simulink model "IL86_NEW_17a"  (R2021b)
settings: Solver=ode1  StartTime=0.0  StopTime=100  FixedStep=0.001  RelTol=1e-3  EnableMultiTasking=on
InitFcn:
  | INIT
values from neighbouring files (symbols this model uses):
  CBN0 = [XB0(1) XB0(2) XB0(3); XB0(4) XB0(5) XB0(6); XB0(7) XB0(8) XB0(9)]    [INIT.m]
  HTR = 500.0    (= 500)    [INIT.m]
  PAR = [1.700E05    5            8.400E06     3.000E07     2.300E07       -0.700E06    0.00E00      0.093E00     0.006E00     0.145E-01       0.586E-01  -0.518E-01    0.876E-01   -1.920E-04    8.110E-05       0.000E00   -2.330E-03    5.020E-04   -1.340E-05    0.515E-01      -3.215E-02   5.300E-04   -0.185E-01   -0.465E-01   -1.290E01       -5.000E00   -0.152E-01   -0.344E-02   -0.064E-02    5.200E-05     ...(+300 chars)    [INITLA.m]
  T_AIL = 1.0/20.2    (= 0.049504950495)    [INITLA.m]
  T_ELEV = 0.1    [INITLA.m]
  T_RUD = 1.0/20.2    (= 0.049504950495)    [INITLA.m]
  T_THROTTLE = 5.0    (= 5)    [INITLA.m]
  TGLIDE = 100.0    (= 100)    [INIT.m]
  THETATR = 0.0    (= 0)    [INIT.m]
  U0_GLIDE = [BAL(1);BAL(3);BAL(4);BAL(5)]    [INIT.m]
  U0_HORIZ = [BAL(1);BAL(3);BAL(4);BAL(5)]    [INIT.m]
  VTR = 80.0    (= 80)    [INIT.m]
  X0 = [Vx1,Vy1,Vz1,Wx1,Wy1,Wz1,GAM,PSI,TET,L,H,Z,FI,LAMD,d,deltaT,deltaV,deltaN,deltaE,Vwx1,Vwy1,Vwz1,HFL,EPS,X1]    [INTSTATE.m]
undefined symbols (not defined in the file or in its folder): BAL
settings Model: Creator=XINGAU  LastModifiedBy=peter
settings SolverCC: AlgebraicLoopSolver=TrustRegion
settings DataIOCC: LimitDataPoints=on  SaveFormat=Array  ReturnWorkspaceOutputs=off
settings OptimizationCC: ExpressionDepthLimit=2147483647  LifeSpan=inf
settings DebuggingCC: UnderspecifiedInitializationDetection=Classic  MergeDetectMultiDrivingBlocksExec=none  SolverPrmCheckMsg=warning  MultiTaskRateTransMsg=warning  StateNameClashWarn=warning  SFUnexpectedBacktrackingDiag=warning  SFNoUnconditionalDefaultTransitionDiag=warning  SFExecutionAtInitializationDiag=none  SFMachineParentedDataDiag=warning  ArithmeticOperatorsInVariantConditions=warning
settings HardwareCC: ProdBitPerPointer=32  ProdBitPerSizeT=32  ProdBitPerPtrDiffT=32  ProdLargestAtomicFloat=None  ProdIntDivRoundTo=Undefined  ProdEndianess=Unspecified  ProdWordSize=32  ProdHWDeviceType=32-bit Generic
settings ModelReferenceCC: PropagateSignalLabelsOutOfModel=off
settings SFSimCC: SimUseLocalCustomCode=off  CustomCodeUndefinedFunction=UseInterfaceOnly
settings RTWCC: RTWUseLocalCustomCode=off
settings CodeAppCC: StateflowObjectComments=on
settings GRTTargetCC: TargetLangStandard=C89/C90 (ANSI)
settings ConfigComp: CovMetricSettings=dw  CovSaveCumulativeToWorkspaceVar=on  CovSaveSingleToWorkspaceVar=on  CovExternalEMLEnable=off

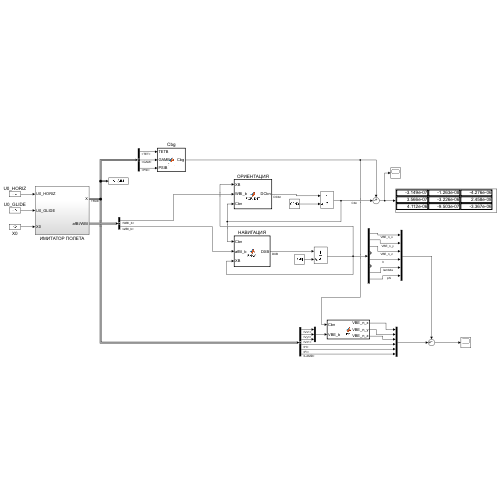
[thumbnail: Simulink's stored preview of the top-level diagram]
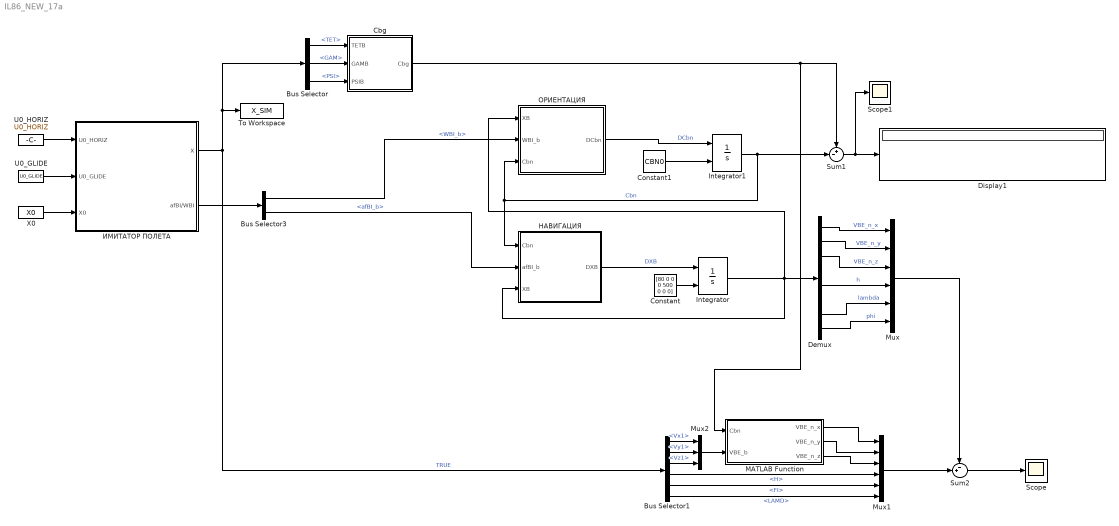
== system IL86_NEW_17a ==
  Bus Selector : BusSelector  OutputSignals=TET,GAM,PSI
  Bus Selector1 : BusSelector  OutputSignals=Vx1,Vy1,Vz1,H,FI,LAMD
  Bus Selector3 : BusSelector  OutputSignals=WBI_b,afBI_b
  Cbg : MATLAB Function  TreatAsAtomicUnit=on
  Constant : Constant  Value=[80 0 0 0 500 0 0 0]
  Constant1 : Constant  Value=CBN0
  Demux : Demux  Outputs=8
  Display1 : Display
  Integrator : Integrator  InitialConditionSource=external
  Integrator1 : Integrator  InitialConditionSource=external
  MATLAB Function : MATLAB Function  TreatAsAtomicUnit=on
  Mux : Mux  Inputs=6
  Mux1 : Mux  Inputs=6
  Mux2 : Mux  Inputs=3
  Scope : Scope
  Scope1 : Scope
  Sum1 : Sum  Inputs=+-|
  Sum2 : Sum  Inputs=-+|
  To Workspace : ToWorkspace  VariableName=X_SIM  SaveFormat=Timeseries  SampleTime=-1
  U0_GLIDE : Constant  Value=U0_GLIDE
  U0_HORIZ : Constant  Value=U0_HORIZ
  X0 : Constant  Value=X0
  ИМИТАТОР ПОЛЕТА : Subsystem
  НАВИГАЦИЯ : MATLAB Function  TreatAsAtomicUnit=on
  ОРИЕНТАЦИЯ : MATLAB Function  TreatAsAtomicUnit=on
  wires:
  X0/1 -> ИМИТАТОР ПОЛЕТА/3(X0)
  U0_HORIZ/1 -> ИМИТАТОР ПОЛЕТА/1(U0_HORIZ)
  U0_GLIDE/1 -> ИМИТАТОР ПОЛЕТА/2(U0_GLIDE)
  ИМИТАТОР ПОЛЕТА/1(X) -> Bus Selector1/1, Bus Selector/1, To Workspace/1  "TRUE"
  Bus Selector/1 -> Cbg/1(TETB)  "<TET>"
  Bus Selector/2 -> Cbg/2(GAMB)  "<GAM>"
  Bus Selector/3 -> Cbg/3(PSIB)  "<PSI>"
  ИМИТАТОР ПОЛЕТА/2(afBI/WBI) -> Bus Selector3/1
  Bus Selector3/2 -> НАВИГАЦИЯ/2(afBI_b)  "<afBI_b>"
  НАВИГАЦИЯ/1(DXB) -> Integrator/1  "DXB"
  Constant/1 -> Integrator/2
  Integrator/1 -> НАВИГАЦИЯ/3(XB), Demux/1, ОРИЕНТАЦИЯ/1(XB)
  ОРИЕНТАЦИЯ/1(DCbn) -> Integrator1/1  "DCbn"
  Bus Selector3/1 -> ОРИЕНТАЦИЯ/2(WBI_b)  "<WBI_b>"
  Integrator1/1 -> ОРИЕНТАЦИЯ/3(Cbn), НАВИГАЦИЯ/1(Cbn), Sum1/2  "Cbn"
  Sum1/1 -> Scope1/1, Display1/1
  Constant1/1 -> Integrator1/2
  Cbg/1(Cbg) -> MATLAB Function/1(Cbn), Sum1/1
  Mux1/1 -> Sum2/2
  Mux/1 -> Sum2/1
  Sum2/1 -> Scope/1
  Demux/1 -> Mux/1  "VBE_n_x"
  Demux/2 -> Mux/2  "VBE_n_y"
  Demux/3 -> Mux/3  "VBE_n_z"
  Demux/8 -> Mux/6  "phi"
  Demux/7 -> Mux/5  "lambda"
  Demux/5 -> Mux/4  "h"
  Bus Selector1/4 -> Mux1/4  "<H>"
  Bus Selector1/5 -> Mux1/5  "<FI>"
  Bus Selector1/6 -> Mux1/6  "<LAMD>"
  Bus Selector1/1 -> Mux2/1  "<Vx1>"
  Bus Selector1/2 -> Mux2/2  "<Vy1>"
  Bus Selector1/3 -> Mux2/3  "<Vz1>"
  Mux2/1 -> MATLAB Function/2(VBE_b)
  MATLAB Function/3(VBE_n_z) -> Mux1/3
  MATLAB Function/2(VBE_n_y) -> Mux1/2
  MATLAB Function/1(VBE_n_x) -> Mux1/1

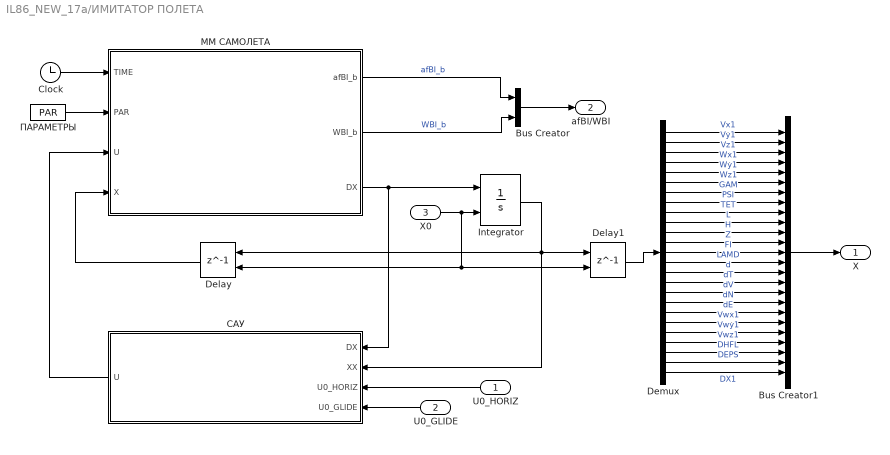
== system IL86_NEW_17a/ИМИТАТОР ПОЛЕТА ==
  U0_HORIZ : Inport
  U0_GLIDE : Inport  Port=2
  X0 : Inport  Port=3
  Bus Creator1 : BusCreator  Inputs=25
  Bus Creator : BusCreator  Inputs=2
  Clock : Clock
  Delay : Delay  DelayLength=1  InitialConditionSource=Input port  InitialCondition=0
      settings: InputPortMap=u0,p4
  Delay1 : Delay  DelayLength=1  InitialConditionSource=Input port  InitialCondition=0
      settings: InputPortMap=u0,p4
  Demux : Demux  Outputs=25
  Integrator : Integrator  InitialConditionSource=external
  ММ САМОЛЕТА : MATLAB Function  TreatAsAtomicUnit=on
  ПАРАМЕТРЫ : Constant  Value=PAR
  САУ : Subsystem
  X : Outport
  afBI/WBI : Outport  Port=2
  wires:
  ПАРАМЕТРЫ/1 -> ММ САМОЛЕТА/2(PAR)
  ММ САМОЛЕТА/3(DX) -> Integrator/1, САУ/1(DX)
  Delay/1 -> ММ САМОЛЕТА/4(X)
  Integrator/1 -> Delay1/1, САУ/2(XX), Delay/1
  ММ САМОЛЕТА/1(afBI_b) -> Bus Creator/1  "afBI_b"
  ММ САМОЛЕТА/2(WBI_b) -> Bus Creator/2  "WBI_b"
  Bus Creator/1 -> afBI/WBI/1
  Demux/1 -> Bus Creator1/1  "Vx1"
  Demux/2 -> Bus Creator1/2  "Vy1"
  Demux/3 -> Bus Creator1/3  "Vz1"
  Demux/4 -> Bus Creator1/4  "Wx1"
  Demux/5 -> Bus Creator1/5  "Wy1"
  Demux/6 -> Bus Creator1/6  "Wz1"
  Demux/7 -> Bus Creator1/7  "GAM"
  Demux/8 -> Bus Creator1/8  "PSI"
  Demux/9 -> Bus Creator1/9  "TET"
  Demux/10 -> Bus Creator1/10  "L"
  Demux/11 -> Bus Creator1/11  "H"
  Demux/12 -> Bus Creator1/12  "Z"
  Demux/13 -> Bus Creator1/13  "FI"
  Demux/14 -> Bus Creator1/14  "LAMD"
  Demux/15 -> Bus Creator1/15  "d"
  Bus Creator1/1 -> X/1
  Demux/16 -> Bus Creator1/16  "dT"
  Demux/17 -> Bus Creator1/17  "dV"
  Demux/18 -> Bus Creator1/18  "dN"
  Demux/19 -> Bus Creator1/19  "dE"
  Demux/20 -> Bus Creator1/20  "Vwx1"
  Demux/21 -> Bus Creator1/21  "Vwy1"
  Clock/1 -> ММ САМОЛЕТА/1(TIME)
  Demux/22 -> Bus Creator1/22  "Vwz1"
  X0/1 -> Delay/2, Delay1/2, Integrator/2
  Demux/23 -> Bus Creator1/23  "DHFL"
  Demux/24 -> Bus Creator1/24  "DEPS"
  Demux/25 -> Bus Creator1/25  "DX1"
  САУ/1(U) -> ММ САМОЛЕТА/3(U)
  U0_HORIZ/1 -> САУ/3(U0_HORIZ)
  U0_GLIDE/1 -> САУ/4(U0_GLIDE)
  Delay1/1 -> Demux/1

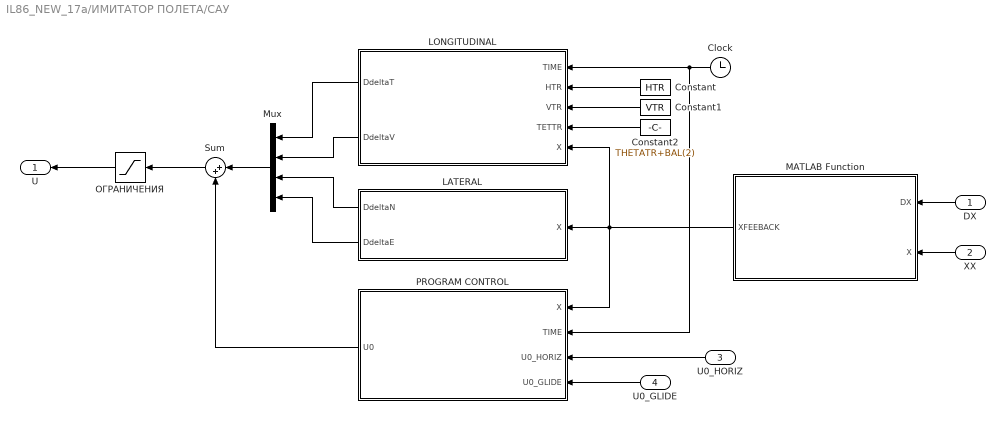
== system IL86_NEW_17a/ИМИТАТОР ПОЛЕТА/САУ ==
  DX : Inport
  XX : Inport  Port=2
  U0_HORIZ : Inport  Port=3
  U0_GLIDE : Inport  Port=4
  Clock : Clock
  Constant : Constant  Value=HTR
  Constant1 : Constant  Value=VTR
  Constant2 : Constant  Value=THETATR+BAL(2)
  LATERAL : MATLAB Function  TreatAsAtomicUnit=on
  LONGITUDINAL : MATLAB Function  TreatAsAtomicUnit=on
  MATLAB Function : MATLAB Function  TreatAsAtomicUnit=on
  Mux : Mux
  PROGRAM CONTROL : MATLAB Function  TreatAsAtomicUnit=on
  Sum : Sum  Inputs=|++
  ОГРАНИЧЕНИЯ : Saturate  UpperLimit=[0.85 30 25 25]  LowerLimit=[0.1 -25 -25 -25]
  U : Outport
  wires:
  Constant/1 -> LONGITUDINAL/2(HTR)
  Constant1/1 -> LONGITUDINAL/3(VTR)
  Constant2/1 -> LONGITUDINAL/4(TETTR)
  Mux/1 -> Sum/1
  Sum/1 -> ОГРАНИЧЕНИЯ/1
  ОГРАНИЧЕНИЯ/1 -> U/1
  LONGITUDINAL/2(DdeltaV) -> Mux/2
  LATERAL/1(DdeltaN) -> Mux/3
  LATERAL/2(DdeltaE) -> Mux/4
  LONGITUDINAL/1(DdeltaT) -> Mux/1
  MATLAB Function/1(XFEEBACK) -> LONGITUDINAL/5(X), PROGRAM CONTROL/1(X), LATERAL/1(X)
  Clock/1 -> LONGITUDINAL/1(TIME), PROGRAM CONTROL/2(TIME)
  PROGRAM CONTROL/1(U0) -> Sum/2
  XX/1 -> MATLAB Function/2(X)
  DX/1 -> MATLAB Function/1(DX)
  U0_HORIZ/1 -> PROGRAM CONTROL/3(U0_HORIZ)
  U0_GLIDE/1 -> PROGRAM CONTROL/4(U0_GLIDE)

== matlab function IL86_NEW_17a/MATLAB Function ==
  data: Cbn input; VBE_b input; VBE_n_x output; VBE_n_y output; VBE_n_z output
function [VBE_n_x,VBE_n_y,VBE_n_z] = fcn(Cbn,VBE_b)
    VBE_n=Cbn*VBE_b;
    VBE_n_x=VBE_n(1);
    VBE_n_y=VBE_n(2);
    VBE_n_z=VBE_n(3);
end

== matlab function IL86_NEW_17a/ИМИТАТОР ПОЛЕТА/ММ САМОЛЕТА ==
  data: TIME input; afBI_b output; WBI_b output; PAR input; U input; X input; DX output; T_THROTTLE parameter; T_ELEV parameter; T_RUD parameter; T_AIL parameter; TGLIDE parameter
function [afBI_b,WBI_b,DX] =FX(TIME,PAR,U,X,T_THROTTLE, T_ELEV, T_RUD, T_AIL,TGLIDE)
    m=PAR(1);
    fiP=PAR(2)*pi/180;
    Jxx=PAR(3);
    Jyy=PAR(4);
    Jzz=PAR(5);
    Jxy=PAR(6);

    Cy0=PAR(7);
    Cy_ALP=PAR(8);
    Cy_deltaV=PAR(9);
    Cy_fi=PAR(10);

    Cx0=PAR(11);
    A=PAR(12);
    B=PAR(13);
    Cx_deltaV=PAR(14);
    Cx_ALP_deltaV=PAR(15);
    Cx_ALP2_deltaV=PAR(16);
    Cx_fi=PAR(17);
    Cx_ALP_fi=PAR(18);
    Cx_ALP2_fi=PAR(19);

    mz0=PAR(20);
    mz_ALP=PAR(21);
    mz_ALP2=PAR(22);
    mz_deltaV=PAR(23);
    mz_fi=PAR(24);
    mz_Wz=PAR(25);
    mz_DALP=PAR(26);        

    Cz_BE=PAR(27);
    Cz_deltaN=PAR(28);

    mx_deltaN=PAR(29);
    mx_ALP_deltaN=PAR(30);
    mx_BE=PAR(31);
    mx_ALP_BE=PAR(32);
    mx_deltaE=PAR(33);
    mx_Wx=PAR(34);
    mx_ALP_Wx=PAR(35);
    mx_ALP2_Wx=PAR(36);
    mx_Wy=PAR(37);
    mx_ALP_Wy=PAR(38);

    my_BE=PAR(39);
    my_deltaN=PAR(40);
    my_Wx=PAR(41);
    my_ALP_Wx=PAR(42);
    my_ALP2_Wx=PAR(43);
    my_Wy=PAR(44);
    my_ALP_Wy=PAR(45);
    my_ALP2_Wy=PAR(46);
    my_DBE=PAR(47);

    xT=PAR(48);
    S=PAR(49);
    l=PAR(50);
    ba=PAR(51);
    fiST=PAR(52);
    ALPKR=PAR(53);
    GR=180.0/pi;
    R00=0.125;    
    PMAX=260000.0;    
    a=6378245.0;
    b=6356856.0;
    e2=(a^2-b^2)/a^2;
    Ue=7292115.0E-11;
    
    % Текущее состоояние
    Vx1=X(1);   Vy1=X(2);    Vz1=X(3);  % Земная скорость в ССК
    Wx1=X(4);   Wy1=X(5);    Wz1=X(6);  % Угловая скорость в ССК
    GAM=X(7);   PSI=X(8);    TET=X(9);  % Углы ориентации в ГСК
    Xg=X(10);   H=X(11);     Zg=X(12);  % Координаты в ГСК
    FI=X(13);   LAMD=X(14);             % Географические углы ориентации
    Vwx1=X(20); Vwy1=X(21);  Vwz1=X(22);% Скорость ветра в ССК 
    % Текущее положение органов управления
    deltaT=X(16);
    deltaV=X(17);
    deltaN=X(18);
    deltaE=X(19);
    % Матрица перехода от ГСК в ССК
    [Cgb] = C_gb(TET, GAM, PSI);

    % Модель гравитации и поля силы тяжести
    [Gg,GTg] = GRAVITY(FI,LAMD,H);  
    Gb=Cgb*Gg;
    % Воздушная скорость ЛА
    Vax1=Vx1-Vwx1;
    Vay1=Vy1-Vwy1;
    Vaz1=Vz1-Vwz1;
    Va=sqrt(Vax1^2+Vay1^2+Vaz1^2);
    ALPHA=-atan(Vay1/Vax1);
    BETA=asin(Vaz1/Va);
    % Перевод в градусы (для аэродинамики)
    ALP=ALPHA*GR+ALPKR;
    BE=BETA*GR;
    % Коэффициенты аэросил
    Cy=Cy0+Cy_ALP*ALP+Cy_deltaV*deltaV+Cy_fi*fiST;
    Cx=Cx0+A*Cy+B*Cy^2+(Cx_deltaV+Cx_ALP_deltaV*ALP+Cx_ALP2_deltaV*ALP^2)*deltaV+...	
		+(Cx_fi+Cx_ALP_fi*ALP+Cx_ALP2_fi*ALP^2)*fiST;
    Cz=Cz_BE*BE+Cz_deltaN*deltaN;
    % Скоростной напор           
    RHO =R00*((288.16-0.0066*H)/288.16)^4.255;
    V=sqrt(Vx1^2+Vy1^2+Vz1^2);
    q=0.5*RHO*V^2*S*norm(GTg);
    % Аэросилы в ЭСК
    Fx=Cx*q;
    Fy=Cy*q;
    Fz=Cz*q;
    % Аэросилы в ССК
    Fx1=Fx*cos(ALPHA)-Fy*sin(ALPHA);
    Fy1=Fx*sin(ALPHA)+Fy*cos(ALPHA);
    Fz1=Fz;   
    % Тяга
    P = deltaT*PMAX*(RHO/R00)^0.75;
    % Вектор абсолютной угловой скорости вращения Земли в ГСК
    WEI_g=[Ue*cos(FI);Ue*sin(FI);0];
    % Вектор абсолютной угловой скорости вращения Земли в ССК
    WEI_b=Cgb*WEI_g;
    % Вектор абсолютной угловой скорости вращения ССК в ССК
    WBI_b=[Wx1;Wy1;Wz1];
    % Вектор земной скорости в ССК
    VBE_b=[Vx1;Vy1;Vz1];
    % Радиус вектор в ГСК
    SINFI=sin(FI);
    chi=sqrt(1-e2*SINFI^2);
    R1=(a+H)/chi;
    R2=(a+H)*(1-e2)/chi^3; 
    rg=[-R1*e2*sin(FI)*cos(FI);R1*(1-e2*(sin(FI))^2);0];
    % Переносное ускорение в ГСК
    APg=-cross(WEI_g,cross(WEI_g,rg));
    % Переносное ускорение в CСК
    APb=Cgb*APg;
    % Кориолисово ускорение в CСК
    AKb=-2*cross(WEI_b,VBE_b);
    % Вектор угловой скорости вращения ССК отн Земли в ССК
    WBE_b=WBI_b-WEI_b;
    % Вспомагательный массив ATemp
    ATb=-cross(WBE_b,VBE_b);
    % Динамика центра масс ЛА    
    dVx1=(1.0/m)*(P*cos(fiP)-Fx1)+APb(1)+AKb(1)+ATb(1)+Gb(1);
    dVy1=(1.0/m)*(P*sin(fiP)+Fy1)+APb(2)+AKb(2)+ATb(2)+Gb(2);
    dVz1=Fz1/m+APb(3)++ATb(3)+Gb(3);

    % Производные от аэродинамических углов
    dALP=-(dVy1*Vax1-dVx1*Vay1)/(Vax1^2+Vay1^2);
    dBE=(dVz1*(Vax1^2+Vay1^2+Vaz1^2)-Vz1*(Vax1*dVx1+Vay1*dVy1+Vaz1*dVz1))/(sqrt(Vax1^2+Vay1^2)*(Vax1^2+Vay1^2+Vaz1^2));
        
    % Текущие угловые скорости в ЭСК
    OMGx=WBE_b(1)*cos(ALPHA)-WBE_b(2)*sin(ALPHA);
    OMGy=WBE_b(1)*sin(ALPHA)+WBE_b(2)*cos(ALPHA);
    OMGz=WBE_b(3); 
    
    % Коэффициенты аэромоментов
    mx=(mx_deltaN+mx_ALP_deltaN*ALP)*deltaN+(mx_BE+mx_ALP_BE*ALP)*BE+mx_deltaE*deltaE+...
        +(mx_Wx+mx_ALP_Wx*ALP+mx_ALP2_Wx*ALP^2)*OMGx*l/(2.0*V)+(mx_Wy+mx_ALP_Wy*ALP)*OMGy*l/(2.0*V);
    my=my_BE*BE+my_deltaN*deltaN+(my_Wx+my_ALP_Wx*ALP+my_ALP2_Wx*ALP^2)*OMGx*l/(2.0*V)+...
        +(my_Wy+my_ALP_Wy*ALP+my_ALP2_Wy*ALP^2)*OMGy*l/(2.0*V)+my_DBE*dBE*l/(2.0*V);
    mz=mz0+mz_ALP*ALP+mz_ALP2*ALP^2+mz_deltaV*deltaV+mz_fi*fiST+mz_Wz*OMGz*ba/V+mz_DALP*dALP*ba/V+(xT-25.0)*Cy*0.01;
    % Аэромоменты в ЭСК
    Mx=mx*q*l;
    My=my*q*l;
    Mz=mz*q*ba;
    % Аэромоменты в ССК   
    Mx1=Mx*cos(ALPHA)+My*sin(ALPHA);
    My1=-Mx*sin(ALPHA)+My*cos(ALPHA);
    Mz1=Mz;
    
    % Угловые ускорения в ССК
    DWx1=(Jyy*Mx1+Jxy*My1+Jxy*(Jxx+Jyy-Jzz)*Wx1*Wz1+(Jyy^2-Jyy*Jzz+Jxy^2)*Wy1*Wz1)/(Jxx*Jyy-Jxy^2);
    DWy1=(Jxy*Mx1+Jxx*My1-(Jxx^2-Jxx*Jzz+Jxy^2)*Wx1*Wz1+Jxy*(Jxx+Jyy-Jzz)*Wy1*Wz1)/(Jxx*Jyy-Jxy^2);
    DWz1=(Mz1-(Jyy-Jxx)*Wx1*Wy1-Jxy*(Wy1^2-Wx1^2))/Jzz;
    
    % Скорость ЛА в ГСК
    DXg=Vx1*cos(PSI)*cos(TET)-Vy1*(cos(PSI)*sin(TET)*cos(GAM)-sin(PSI)*sin(GAM))+Vz1*(sin(PSI)*cos(GAM)+cos(PSI)*sin(TET)*sin(GAM));
    DH=Vx1*sin(TET)+Vy1*cos(TET)*cos(GAM)-Vz1*cos(TET)*sin(GAM);
    DZg=-Vx1*sin(PSI)*cos(TET)+Vy1*(cos(PSI)*sin(GAM)+sin(PSI)*sin(TET)*cos(GAM))+Vz1*(cos(PSI)*cos(GAM)-sin(PSI)*sin(TET)*sin(GAM));
    
    % Вектор угловой скорости вращения ГСК отн. Земли в ГСК
    WGE_g=[DZg/R1; DZg*tan(FI)/R1; -DXg/R2];
    % Вектор абсолютной угловой скорости вращения ГСК в ГСК
    WGI_g=WGE_g+WEI_g;    
    % Вектор абсолютной угловой скорости ГСК в ССК
    WGI_b=Cgb*WGI_g;
    
    % Вектор угловой скорости ЛА отн ГСК в ССК
    WBG_b = WBI_b - WGI_b;
%     P = WBI_b(1) - WGI_b(1);
%     R = WBI_b(2) - WGI_b(2);
%     Q = WBI_b(3) - WGI_b(3);

    % Производные от углов ориентации
    DPSI   = (WBG_b(2)*cos(GAM) - WBG_b(3)*sin(GAM)) / cos(TET);
    DTET   =  WBG_b(3)*cos(GAM) + WBG_b(2)*sin(GAM);
    DGAM   =  WBG_b(1) - DPSI*sin(TET);
    
    % Производные от географических углов ориентации
    DFI=DXg/R2;
    DLAMD=DZg/R1/cos(FI);
    
    Dd=0.0;
    if (TIME>TGLIDE)
        THETA=asin(DH/sqrt(DXg^2+DZg^2));
        THETATR=-3.0*pi/180.0;
        Dd = V * sin(THETA - THETATR);
    end
    
    % Производные от скоростей ветра
    DVwx1=0.0;
    DVwy1=0.0;
    DVwz1=0.0;
    
    % Органы управления
    DdeltaT=(U(1)-deltaT)/T_THROTTLE;
	DdeltaV=(U(2)-deltaV)/T_ELEV;
	DdeltaN=(U(3)-deltaN)/T_RUD;
	DdeltaE=(U(4)-deltaE)/T_AIL;
    
    % В режиме выравнивании
    DHFL=0.0;DEPS=0.0;DX1=0.0;
    if (H<=15.0)
        DHFL=-0.5*X(23);
        DEPS=X(23)-H;
        DX1=-10.0*X(25)+X(24);
    end
    
    % Вектор правой части системы диффур. движения ЛА
    DX=[dVx1,dVy1,dVz1,...
        DWx1,DWy1,DWz1,...
        DGAM,DPSI,DTET,...
        DXg,DH,DZg,...
        DFI,DLAMD,...
        Dd,...
        DdeltaT,DdeltaV,DdeltaN,DdeltaE,...
        DVwx1,DVwy1,DVwz1,...
        DHFL,DEPS,DX1]'; 
    
    % Для БИНС
    axb=(1.0/m)*(P*cos(fiP)-Fx1);
    ayb=(1.0/m)*(P*sin(fiP)+Fy1);
    azb=Fz1/m;
    afBI_b=[axb;ayb;azb];    
    
end

function [Gg,GTg] = GRAVITY(FI,LAMD,H)    
    %% Параметры гравитационного поля Земли
    d00=39861679.0E+7;
    d20=175519.0E+20;
    Ue=7292115.0E-11;
    a=6378245.0;
    b=6356856.0;
    e2=(a^2-b^2)/a^2;

    %% Геоцентрическая широта
    SINFI=sin(FI);
    SINMU=e2*SINFI*cos(FI)/sqrt(1-(2*e2-e2^2)*SINFI^2);
    COSMU=(1-e2*SINFI^2)/sqrt(1-(2*e2-e2^2)*SINFI^2);
    MU=asin(SINMU);
    FIe=FI-MU;

    %% Геоцентрический радиус-вектор
    chi=sqrt(1-e2*SINFI^2);
    Xe=(a+H)/chi*cos(FI)*sin(LAMD);
    Ye=(a+H)*(1-e2)/chi*SINFI;
    Ze=(a+H)/chi*cos(FI)*cos(LAMD);
    r=sqrt(Xe^2+Ye^2+Ze^2);

    %% Проекции вектора гравитационного ускорения на местной вертикаль и перпендикулярную к ней ось
    Gr=-d00/(r^2)-3/2*d20/(r^4)*(3*sin(FIe)*sin(FIe)-1);
    Gfie=-3/2*d20/(r^4)*sin(2*FIe);

    Gn=Gr*COSMU+Gfie*SINMU;
    Gfi=-Gr*SINMU+Gfie*COSMU; 
    
%     if (FLATEARTH==1)
%         Ue=0.0;
%         Gfi=0.0;
%     end
    
    %% Гравитационное ускорение в ГСК
    Gg=[Gfi;Gn;0];
    
    %% Ускорение силы тяжести в ГСК
    GTn=Gn-r*Ue^2*cos(FIe)*cos(FI);
    GTfi=Gfi+r*Ue^2*cos(FIe)*SINFI;%должна быть равна 0

    GTg=[0;GTn;0];
end

%% МАТРИЦЫ ПЕРЕХОДОВ
% 1. Переход от ГСК в ССК
function [Cgb] = C_gb(TET, PH, PSI)

Cgb = zeros(3,3);

Cgb(1,1) =  cos(PSI) * cos(TET);
Cgb(1,2) =  sin(TET);
Cgb(1,3) = -sin(PSI) * cos(TET);

Cgb(2,1) = -cos(PSI)*sin(TET)*cos(PH)+sin(PSI)*sin(PH);
Cgb(2,2) =  cos(TET)*cos(PH);
Cgb(2,3) =  cos(PSI)*sin(PH)+sin(PSI)*sin(TET)*cos(PH);

Cgb(3,1) =  cos(PSI)*sin(TET)*sin(PH)+sin(PSI)*cos(PH);
Cgb(3,2) = -cos(TET)*sin(PH);
Cgb(3,3) =  cos(PSI)*cos(PH)-sin(PSI)*sin(TET)*sin(PH); 
end

== matlab function IL86_NEW_17a/НАВИГАЦИЯ ==
  data: Cbn input; afBI_b input; XB input; DXB output
function DXB = FNAVI(Cbn, afBI_b, XB)
    %% константы
    a=6378245.0;
    b=6356856.0;
    omega_e=7292115e-11;
    e=sqrt(1-(b^2)/(a^2));
    d_00=39861679e7;
    d_20=175519e+20;
    x=1;
    y=2;
    z=3;
    %%
    afBI_n=Cbn*afBI_b;
    VBE_n=[XB(1);
                    XB(2);
                    XB(3)];
    h=XB(5);
    lambda=XB(7);
    phi=XB(8);
    Cen=[-sin(phi)*sin(lambda) cos(phi) -sin(phi)*cos(lambda);
                cos(phi)*sin(lambda) sin(phi) cos(phi)*cos(lambda);
                cos(lambda) 0 -sin(lambda)];
    WEI_e=[0 omega_e 0]';
    WEI_n=Cen*WEI_e;
    chi=sqrt(1-e^2*(sin(phi))^2);
    r_1=(a+h)/chi;
    r_2=(a+h)*(1-e^2)/chi^3;
    WNE_n=[VBE_n(z)/r_1;
                     VBE_n(z)*tan(phi)/r_1;
                     -VBE_n(x)/r_2];
    mu=asin(e^2*sin(phi)*cos(phi)/sqrt(1-(2*e^2-e^4)*(sin(phi))^2));
    phi_e=phi-mu;
    r_e=(a+h)/chi*[cos(phi)*sin(lambda); 
        (1-e^2)*sin(phi); 
        cos(phi)*cos(lambda)];
    r_n=Cen*r_e;
    r=sqrt((r_n(x))^2+(r_n(y))^2+(r_n(z))^2);
    g_r=-d_00/r^2-3*d_20*(2*(sin(phi))^2-1)/(2*r^4);
    g_phi_e=3*d_20*sin(2*phi_e)/(2*r^4);
    g_n=[-g_r*sin(mu)+g_phi_e*cos(mu);
             g_r*cos(mu)+g_phi_e*sin(mu);
             0];
    DVBE_n=afBI_n-cross(2*WEI_n, VBE_n)-(cross(WNE_n,VBE_n)+cross(WEI_n,cross(WEI_n,r_n)))+g_n;
    Dx_g=VBE_n(x);
    Dh=VBE_n(y);
    Dz_g=VBE_n(z);
    Dlambda=VBE_n(x)/(r_1*cos(phi));
    Dphi=-VBE_n(z)/r_2;
    DXB=[DVBE_n;
                Dx_g;
                Dh;
                Dz_g;
                Dlambda;
                Dphi];
end

== matlab function IL86_NEW_17a/Cbg ==
  data: TETB input; GAMB input; PSIB input; Cbg output
function Cbg   = C_gb(TETB, GAMB, PSIB)

Cbg = zeros(3,3);

Cbg(1,1)=cos(PSIB)*cos(TETB);
Cbg(1,2)=-cos(PSIB)*sin(TETB)*cos(GAMB)+sin(PSIB)*sin(GAMB);
Cbg(1,3)=cos(PSIB)*sin(TETB)*sin(GAMB)+sin(PSIB)*cos(GAMB);

Cbg(2,1)=sin(TETB);
Cbg(2,2)=cos(TETB)*cos(GAMB);
Cbg(2,3)=-cos(TETB)*sin(GAMB);

Cbg(3,1)=-cos(TETB)*sin(PSIB);	
Cbg(3,2)=cos(PSIB)*sin(GAMB)+sin(PSIB)*sin(TETB)*cos(GAMB);	
Cbg(3,3)=cos(PSIB)*cos(GAMB)-sin(PSIB)*sin(TETB)*sin(GAMB);
end

== matlab function IL86_NEW_17a/ИМИТАТОР ПОЛЕТА/САУ/LATERAL ==
  data: X input; DdeltaN output; DdeltaE output
function [DdeltaN,DdeltaE] = AUTOPILOT_LAT(X)
%    Wx=X(1); GAM=X(5); Az=X(9); Vz=X(12); Z=X(15);
%    Wy=X(2); PSI=X(6);

    Wx=X(1);    Wy=X(2);
    GAM=X(4);   PSI=X(5);
    Az=X(7);
    Vz=X(8);
    Z=X(9);


    K_AIL_Z= -0.007852;
    K_AIL_Vz = 0.008516;
    K_AIL_Az = 0.323961;
    K_AIL_GAM = -0.295147;
    K_AIL_Wx = -4.501701;
    K_RUD_Z = -0.010000;
    K_RUD_Vz = -0.000950;
    K_RUD_Az= 0.049556;
    K_RUD_PSI= -0.124876;
    K_RUD_Wy= 2.706971;
	de=K_AIL_Wx*Wx+K_AIL_GAM*GAM+K_AIL_Az*Az+K_AIL_Vz*Vz+K_AIL_Z*Z/57.3;
	dn=K_RUD_Wy*Wy+K_RUD_PSI*PSI+K_RUD_Az*Az+K_RUD_Vz*Vz+K_RUD_Z*Z/57.3;

	DdeltaN=dn*57.3;
	DdeltaE=de*57.3;
end

== matlab function IL86_NEW_17a/ИМИТАТОР ПОЛЕТА/САУ/LONGITUDINAL ==
  data: TIME input; HTR input; VTR input; TETTR input; X input; DdeltaT output; DdeltaV output; TGLIDE parameter
function [DdeltaT,DdeltaV] = AUTOPILOT_LONG(TIME,HTR,VTR,TETTR,X,TGLIDE)
    %% оценка состояния ЛА
    %H=X(14);
    %V=sqrt(X(1)^2+X(2)^2+X(3)^2);   DV=sqrt(X(7)^2+X(8)^2+X(9)^2);
    %Wz=X(3);    TET=X(4);    
    V=X(10);
    DV=X(11);
    H=X(12);
    Wz=X(3);
    TET=X(6);
    THETA=X(13);
    d=X(14);
    HFL=X(15);
	EPS=X(16);
    X1=X(17);   
    
    %% Правило переключения между режимами
    if (TIME<TGLIDE && H>400)
        KEY=0;
    elseif (H>15.0)
        KEY=1;
    else
        KEY=2;
    end
    
    %% Законы управления
    DdeltaT=0.0;
    DdeltaV=0.0;
    if (KEY==0)
        % коэффициента автопилота
        K_ELEV_W= 1.339591;
        K_ELEV_THETA = -1.332765;
        K_ELEV_H = -0.127573;
        K_THROTTLE_V = 0.145670;
        K_THROTTLE_DV = -0.307940;
        K_ELEV_V = -0.148772;
        K_THROTTLE_H = 0.006174;
        % закон управления	
        DdeltaT = K_THROTTLE_V * (VTR - V) + K_THROTTLE_DV * DV+K_THROTTLE_H*(HTR - H);
        DdeltaV = K_ELEV_W * Wz * 57.3 + K_ELEV_THETA * (TETTR-TET)*57.3 + K_ELEV_H*(HTR - H)+ K_ELEV_V*(VTR - V);
    end
    if (KEY==1)
        THETATR=-3.0*pi/180;
        % коэффициента автопилота
        K_ELEV_W= 16.714542;
         K_ELEV_THETA = -5.069737;
         K_ELEV_d = 0.472349;
         K_THROTTLE_V = 1.124095;
         K_THROTTLE_DV = -12.788234;
         K_ELEV_V = 1.264112;
        % закон управления
        DdeltaT = K_THROTTLE_V * (VTR - V) + K_THROTTLE_DV * DV;
        DdeltaV = K_ELEV_W * Wz * 57.3 + K_ELEV_THETA * (THETATR-THETA)*57.3 + K_ELEV_d*d+ K_ELEV_V*(VTR - V);    
    end
    if (KEY==2)        
        k1= -918.800309;
        k2 = 999.988246;
        k3 = -116.617694;
        k4 = -6.636565;
        k5 = 77.282784;
        k6 = 0.054131;
        DdeltaV=10*k1*X1+k2*EPS+k3*(HFL-H)+k4*THETA*57.3+k5*Wz*57.3+k6*HFL;
    end
end

== matlab function IL86_NEW_17a/ОРИЕНТАЦИЯ ==
  data: XB input; WBI_b input; Cbn input; DCbn output
function DCbn   =FORIENT(XB,WBI_b,Cbn)
    %% константы
    a=6378245;
    b=6356856;
    omega_e=7292115e-11;
    e=sqrt(1-(b^2)/(a^2));
    %d_00=39861679e7;
    %d_20=175519e+20;
    x=1;
    y=2;
    z=3;
    %% вычисления
    skew_matrix_WBI_b=[0 -WBI_b(z) WBI_b(y);
                                          WBI_b(z) 0 -WBI_b(x);
                                          -WBI_b(y) WBI_b(x) 0];
    VBE_n=[XB(1);
                    XB(2);
                    XB(3)];
    h=XB(5);
    lambda=XB(7);
    phi=XB(8);
    CEN=[-sin(phi)*sin(lambda) cos(phi) -sin(phi)*cos(lambda);
                cos(phi)*sin(lambda) sin(phi) cos(phi)*cos(lambda);
                cos(lambda) 0 -sin(lambda)];
    WEI_e=[0 omega_e 0]';
    WEI_n=CEN*WEI_e;
    chi=sqrt(1-e^2*(sin(phi))^2);
    r_1=(a+h)/chi;
    r_2=(a+h)*(1-e^2)/chi^3;
    WNE_n=[VBE_n(z)/r_1;
                     VBE_n(z)*tan(phi)/r_1;
                     -VBE_n(x)/r_2];
    WNI_n=WNE_n+WEI_n;
    skew_matrix_WNI_n=[0 -WNI_n(z) WNI_n(y);
                                          WNI_n(z) 0 -WNI_n(x);
                                          -WNI_n(y) WNI_n(x) 0];
    DCbn=Cbn*skew_matrix_WBI_b-skew_matrix_WNI_n*Cbn;
end

== matlab function IL86_NEW_17a/ИМИТАТОР ПОЛЕТА/САУ/MATLAB Function ==
  data: DX input; X input; XFEEBACK output
function XFEEBACK  = fcn(DX,X)
Wx=X(4);    Wy=X(5);    Wz=X(6);
GAM=X(7);   PSI=X(8);   TET=X(9);
V=sqrt(X(1)^2+X(2)^2+X(3)^2);
DV=sqrt(DX(1)^2+DX(2)^2+DX(3)^2);
H=X(11); 
Z=X(12);
Az=DX(3);
Vxg=DX(10);
Vyg=DX(11);
Vzg=DX(12);
d=X(15); 
THETA=asin(Vyg/sqrt(Vxg^2+Vzg^2));
HFL=X(23);
EPS=X(24);
X1=X(25);
XFEEBACK=[Wx Wy Wz GAM PSI TET Az Vzg Z V DV H THETA d HFL EPS X1];

== matlab function IL86_NEW_17a/ИМИТАТОР ПОЛЕТА/САУ/PROGRAM CONTROL ==
  data: X input; TIME input; U0 output; U0_HORIZ input; U0_GLIDE input; TGLIDE parameter
function U0 = PROGCNTRL(X,TIME,U0_HORIZ,U0_GLIDE,TGLIDE)
    U0=[0;0;0;0];
    %% Текущая высота
    H=X(12);
    %% Время отсчитанное от начала выравнивания	
    TFLARE=0.0; %(ошибка!!!)
    DT=1.E-3;    
    %% Правило переключения между режимами
    if (TIME<TGLIDE && H>400)
        KEY=0;
    elseif (H>15.0)
        KEY=1;
    else
        KEY=2;
    end
    %% Законы управления
    if (KEY==0)
        U0=U0_HORIZ;
    end
    if (KEY==1)
        U0=U0_GLIDE;
    end
    if (KEY==2)
        TFLARE=TFLARE+DT; 
        DRGR_BAL=U0_GLIDE(1);
        if (TFLARE<=5.0)
			deltaDT=DRGR_BAL-(DRGR_BAL-0.1)/5.0*TFLARE;
		else
			deltaDT=0.1;
        end
        U0=[deltaDT;U0_GLIDE(2);U0_GLIDE(3);U0_GLIDE(4)];
    end
end
